simulink model "rate_change_filters_txrx_2ch"  (Simulink 7.7)
settings: Solver=VariableStepDiscrete  SolverMode=SingleTasking  StartTime=0.0  StopTime=1e3  RelTol=1e-3
InitFcn:
  | rate_change_filters_init
StartFcn:
  | rate_change_filters_init
values from neighbouring files (symbols this model uses):
  h32_rs = h32    [rate_change_filters_init.m]
  h64_rs = permute(reshape(h64(1:64),4,4,4),[2 1 3])    [rate_change_filters_init.m]
undefined symbols (not defined in the file or in its folder): gcbh, xlBlockLoadCallback, xlGetNormalizedPeriod
libraries: xbsIndex_r4 x499, simulink x8
(part 3 of 3)

== system rate_change_filters_txrx_2ch/Tx Path/2-Ch Interp A/Adders ==
  In1 : Inport
  In2 : Inport  Port=2
  In3 : Inport  Port=3
  In4 : Inport  Port=4
  In5 : Inport  Port=5
  In6 : Inport  Port=6
  In7 : Inport  Port=7
  In8 : Inport  Port=8
  AddSub{1,3..4,7} (4 alike) : xbsIndex_r4/AddSub  mode=Addition  use_carryin=off  use_carryout=off  en=off  latency=0  precision=Full  arith_type=Unsigned  n_bits=16  bin_pt=14  quantization=Truncate  overflow=Wrap  dbl_ovrd=off  use_behavioral_HDL=off  hw_selection=Fabric  pipelined=off  use_rpm=on  block_type=addsub
      settings: xl_area=[10 0 0 18 0 0 0]  block_version=10.1.3
  AddSub2 : xbsIndex_r4/AddSub  mode=Addition  use_carryin=off  use_carryout=off  en=off  latency=1  precision=Full  arith_type=Unsigned  n_bits=16  bin_pt=14  quantization=Truncate  overflow=Wrap  dbl_ovrd=off  use_behavioral_HDL=off  hw_selection=Fabric  pipelined=off  use_rpm=on  block_type=addsub
      settings: xl_area=[10 20 0 19 0 0 0]  block_version=10.1.3
  AddSub5 : xbsIndex_r4/AddSub  mode=Addition  use_carryin=off  use_carryout=off  en=off  latency=1  precision=Full  arith_type=Unsigned  n_bits=16  bin_pt=14  quantization=Truncate  overflow=Wrap  dbl_ovrd=off  use_behavioral_HDL=off  hw_selection=Fabric  pipelined=off  use_rpm=on  block_type=addsub
      settings: xl_area=[10 20 0 19 0 0 0]  block_version=10.1.3
  AddSub8 : xbsIndex_r4/AddSub  mode=Addition  use_carryin=off  use_carryout=off  en=off  latency=0  precision=User Defined  arith_type="Signed  (2's comp)"  n_bits=16  bin_pt=15  quantization=Truncate  overflow=Flag as error  dbl_ovrd=off  use_behavioral_HDL=off  hw_selection=Fabric  pipelined=off  use_rpm=on  block_type=addsub
      settings: xl_area=[11 0 0 20 0 0 0]  block_version=10.1.3
  Out1 : Outport
  wires:
  AddSub5/1 -> AddSub8/2
  AddSub2/1 -> AddSub8/1
  AddSub4/1 -> AddSub5/2
  AddSub3/1 -> AddSub5/1
  AddSub1/1 -> AddSub2/2
  AddSub7/1 -> AddSub2/1
  In1/1 -> AddSub7/1
  In2/1 -> AddSub7/2
  In3/1 -> AddSub1/1
  In4/1 -> AddSub1/2
  AddSub8/1 -> Out1/1
  In5/1 -> AddSub3/1
  In6/1 -> AddSub3/2
  In7/1 -> AddSub4/1
  In8/1 -> AddSub4/2

== system rate_change_filters_txrx_2ch/Tx Path/2-Ch Interp A/Mults & ROMs ==
  In1 : Inport
  In2 : Inport  Port=2
  In3 : Inport  Port=3
  In4 : Inport  Port=4
  In5 : Inport  Port=5
  In6 : Inport  Port=6
  In7 : Inport  Port=7
  In8 : Inport  Port=8
  Mult{1..8} (8 alike) : xbsIndex_r4/Mult  precision=User Defined  arith_type="Signed  (2's comp)"  n_bits=18  bin_pt=17  quantization=Truncate  overflow=Flag as error  en=off  latency=1  dbl_ovrd=off  use_behavioral_HDL=off  opt=Speed  use_embedded=on  optimum_pipeline=off  pipeline=on  use_rpm=on  placement_style=Triangular  block_type=mult
      settings: infoedit=Hardware notes: To use the internal pipeline stage of the dedicated multiplier you must select 'Pipeline for maximum performance'.  xl_area=[9 -15 0 18 0 1 0]  block_version=10.1.3
  Out1 : Outport
  Out2 : Outport  Port=2
  Out3 : Outport  Port=3
  Out4 : Outport  Port=4
  Out5 : Outport  Port=5
  Out6 : Outport  Port=6
  Out7 : Outport  Port=7
  Out8 : Outport  Port=8
  wires:
  [TX_ROM_7] -> Mult8/2
  [TX_ROM_6] -> Mult7/2
  [TX_ROM_5] -> Mult6/2
  [TX_ROM_4] -> Mult5/2
  [TX_ROM_3] -> Mult4/2
  [TX_ROM_2] -> Mult3/2
  [TX_ROM_1] -> Mult1/2
  [TX_ROM_0] -> Mult2/2
  In1/1 -> Mult2/1
  Mult2/1 -> Out1/1
  In2/1 -> Mult1/1
  Mult1/1 -> Out2/1
  In3/1 -> Mult3/1
  Mult3/1 -> Out3/1
  In4/1 -> Mult4/1
  Mult4/1 -> Out4/1
  In5/1 -> Mult5/1
  Mult5/1 -> Out5/1
  In6/1 -> Mult6/1
  Mult6/1 -> Out6/1
  In7/1 -> Mult7/1
  Mult7/1 -> Out7/1
  In8/1 -> Mult8/1
  Mult8/1 -> Out8/1

== system rate_change_filters_txrx_2ch/Tx Path/2-Ch Interp A/Sample RAMs ==
  A : Inport
  B : Inport  Port=2
  Delays : Subsystem
  Delays1 : Subsystem
  Time Division Multiplexer{1..7,16} (8 alike) : xbsIndex_r4/Time Division Multiplexer  inputs=2  vin=off  dbl_ovrd=off  explicit_period=off  period=1  block_type=tdm
      settings: infoedit="Multiple inputs are sampled and  presented serially at the output."  xl_area=[3 2 0 35 0 0 0]  block_version=10.1.3
  Out1 : Outport
  Out2 : Outport  Port=2
  Out3 : Outport  Port=3
  Out4 : Outport  Port=4
  Out5 : Outport  Port=5
  Out6 : Outport  Port=6
  Out7 : Outport  Port=7
  Out8 : Outport  Port=8
  wires:
  Delays/1(Out1) -> Time Division Multiplexer16/1
  Delays1/1(Out1) -> Time Division Multiplexer16/2
  Delays/2(Out2) -> Time Division Multiplexer1/1
  Delays1/2(Out2) -> Time Division Multiplexer1/2
  Delays/3(Out3) -> Time Division Multiplexer3/1
  Delays/4(Out4) -> Time Division Multiplexer2/1
  Delays/5(Out5) -> Time Division Multiplexer5/1
  Delays/6(Out6) -> Time Division Multiplexer4/1
  Delays/7(Out7) -> Time Division Multiplexer7/1
  Delays/8(Out8) -> Time Division Multiplexer6/1
  Delays1/3(Out3) -> Time Division Multiplexer3/2
  Delays1/4(Out4) -> Time Division Multiplexer2/2
  Delays1/5(Out5) -> Time Division Multiplexer5/2
  Delays1/6(Out6) -> Time Division Multiplexer4/2
  Delays1/7(Out7) -> Time Division Multiplexer7/2
  Delays1/8(Out8) -> Time Division Multiplexer6/2
  Time Division Multiplexer16/1 -> Out1/1
  Time Division Multiplexer1/1 -> Out2/1
  Time Division Multiplexer3/1 -> Out3/1
  Time Division Multiplexer2/1 -> Out4/1
  A/1 -> Delays/1(X)
  Time Division Multiplexer5/1 -> Out5/1
  Time Division Multiplexer4/1 -> Out6/1
  Time Division Multiplexer7/1 -> Out7/1
  Time Division Multiplexer6/1 -> Out8/1
  B/1 -> Delays1/1(X)

== system rate_change_filters_txrx_2ch/Tx Path/2-Ch Interp B/Adders ==
  In1 : Inport
  In2 : Inport  Port=2
  In3 : Inport  Port=3
  In4 : Inport  Port=4
  In5 : Inport  Port=5
  In6 : Inport  Port=6
  In7 : Inport  Port=7
  In8 : Inport  Port=8
  AddSub{1,3..4,7} (4 alike) : xbsIndex_r4/AddSub  mode=Addition  use_carryin=off  use_carryout=off  en=off  latency=0  precision=Full  arith_type=Unsigned  n_bits=16  bin_pt=14  quantization=Truncate  overflow=Wrap  dbl_ovrd=off  use_behavioral_HDL=off  hw_selection=Fabric  pipelined=off  use_rpm=on  block_type=addsub
      settings: xl_area=[10 0 0 18 0 0 0]  block_version=10.1.3
  AddSub2 : xbsIndex_r4/AddSub  mode=Addition  use_carryin=off  use_carryout=off  en=off  latency=1  precision=Full  arith_type=Unsigned  n_bits=16  bin_pt=14  quantization=Truncate  overflow=Wrap  dbl_ovrd=off  use_behavioral_HDL=off  hw_selection=Fabric  pipelined=off  use_rpm=on  block_type=addsub
      settings: xl_area=[10 20 0 19 0 0 0]  block_version=10.1.3
  AddSub5 : xbsIndex_r4/AddSub  mode=Addition  use_carryin=off  use_carryout=off  en=off  latency=1  precision=Full  arith_type=Unsigned  n_bits=16  bin_pt=14  quantization=Truncate  overflow=Wrap  dbl_ovrd=off  use_behavioral_HDL=off  hw_selection=Fabric  pipelined=off  use_rpm=on  block_type=addsub
      settings: xl_area=[10 20 0 19 0 0 0]  block_version=10.1.3
  AddSub8 : xbsIndex_r4/AddSub  mode=Addition  use_carryin=off  use_carryout=off  en=off  latency=0  precision=User Defined  arith_type="Signed  (2's comp)"  n_bits=16  bin_pt=15  quantization=Truncate  overflow=Flag as error  dbl_ovrd=off  use_behavioral_HDL=off  hw_selection=Fabric  pipelined=off  use_rpm=on  block_type=addsub
      settings: xl_area=[11 0 0 20 0 0 0]  block_version=10.1.3
  Out1 : Outport
  wires:
  In8/1 -> AddSub4/2
  In7/1 -> AddSub4/1
  In6/1 -> AddSub3/2
  In5/1 -> AddSub3/1
  AddSub8/1 -> Out1/1
  In4/1 -> AddSub1/2
  In3/1 -> AddSub1/1
  In2/1 -> AddSub7/2
  In1/1 -> AddSub7/1
  AddSub7/1 -> AddSub2/1
  AddSub1/1 -> AddSub2/2
  AddSub3/1 -> AddSub5/1
  AddSub4/1 -> AddSub5/2
  AddSub2/1 -> AddSub8/1
  AddSub5/1 -> AddSub8/2

== system rate_change_filters_txrx_2ch/Tx Path/2-Ch Interp B/Mults & ROMs ==
  In1 : Inport
  In2 : Inport  Port=2
  In3 : Inport  Port=3
  In4 : Inport  Port=4
  In5 : Inport  Port=5
  In6 : Inport  Port=6
  In7 : Inport  Port=7
  In8 : Inport  Port=8
  Mult{1..8} (8 alike) : xbsIndex_r4/Mult  precision=User Defined  arith_type="Signed  (2's comp)"  n_bits=18  bin_pt=17  quantization=Truncate  overflow=Flag as error  en=off  latency=1  dbl_ovrd=off  use_behavioral_HDL=off  opt=Speed  use_embedded=on  optimum_pipeline=off  pipeline=on  use_rpm=on  placement_style=Triangular  block_type=mult
      settings: infoedit=Hardware notes: To use the internal pipeline stage of the dedicated multiplier you must select 'Pipeline for maximum performance'.  xl_area=[9 -15 0 18 0 1 0]  block_version=10.1.3
  Out1 : Outport
  Out2 : Outport  Port=2
  Out3 : Outport  Port=3
  Out4 : Outport  Port=4
  Out5 : Outport  Port=5
  Out6 : Outport  Port=6
  Out7 : Outport  Port=7
  Out8 : Outport  Port=8
  wires:
  Mult8/1 -> Out8/1
  In8/1 -> Mult8/1
  Mult7/1 -> Out7/1
  In7/1 -> Mult7/1
  Mult6/1 -> Out6/1
  In6/1 -> Mult6/1
  Mult5/1 -> Out5/1
  In5/1 -> Mult5/1
  Mult4/1 -> Out4/1
  In4/1 -> Mult4/1
  Mult3/1 -> Out3/1
  In3/1 -> Mult3/1
  Mult1/1 -> Out2/1
  In2/1 -> Mult1/1
  Mult2/1 -> Out1/1
  In1/1 -> Mult2/1
  [TX_ROM_0] -> Mult2/2
  [TX_ROM_1] -> Mult1/2
  [TX_ROM_2] -> Mult3/2
  [TX_ROM_3] -> Mult4/2
  [TX_ROM_4] -> Mult5/2
  [TX_ROM_5] -> Mult6/2
  [TX_ROM_6] -> Mult7/2
  [TX_ROM_7] -> Mult8/2

== system rate_change_filters_txrx_2ch/Tx Path/2-Ch Interp B/Sample RAMs ==
  A : Inport
  B : Inport  Port=2
  Delays : Subsystem
  Delays1 : Subsystem
  Time Division Multiplexer{1..7,16} (8 alike) : xbsIndex_r4/Time Division Multiplexer  inputs=2  vin=off  dbl_ovrd=off  explicit_period=off  period=1  block_type=tdm
      settings: infoedit="Multiple inputs are sampled and  presented serially at the output."  xl_area=[3 2 0 35 0 0 0]  block_version=10.1.3
  Out1 : Outport
  Out2 : Outport  Port=2
  Out3 : Outport  Port=3
  Out4 : Outport  Port=4
  Out5 : Outport  Port=5
  Out6 : Outport  Port=6
  Out7 : Outport  Port=7
  Out8 : Outport  Port=8
  wires:
  B/1 -> Delays1/1(X)
  Time Division Multiplexer6/1 -> Out8/1
  Time Division Multiplexer7/1 -> Out7/1
  Time Division Multiplexer4/1 -> Out6/1
  Time Division Multiplexer5/1 -> Out5/1
  A/1 -> Delays/1(X)
  Time Division Multiplexer2/1 -> Out4/1
  Time Division Multiplexer3/1 -> Out3/1
  Time Division Multiplexer1/1 -> Out2/1
  Time Division Multiplexer16/1 -> Out1/1
  Delays1/8(Out8) -> Time Division Multiplexer6/2
  Delays1/7(Out7) -> Time Division Multiplexer7/2
  Delays1/6(Out6) -> Time Division Multiplexer4/2
  Delays1/5(Out5) -> Time Division Multiplexer5/2
  Delays1/4(Out4) -> Time Division Multiplexer2/2
  Delays1/3(Out3) -> Time Division Multiplexer3/2
  Delays/8(Out8) -> Time Division Multiplexer6/1
  Delays/7(Out7) -> Time Division Multiplexer7/1
  Delays/6(Out6) -> Time Division Multiplexer4/1
  Delays/5(Out5) -> Time Division Multiplexer5/1
  Delays/4(Out4) -> Time Division Multiplexer2/1
  Delays/3(Out3) -> Time Division Multiplexer3/1
  Delays1/2(Out2) -> Time Division Multiplexer1/2
  Delays/2(Out2) -> Time Division Multiplexer1/1
  Delays1/1(Out1) -> Time Division Multiplexer16/2
  Delays/1(Out1) -> Time Division Multiplexer16/1

== system rate_change_filters_txrx_2ch/Rx Path/2-Ch Decimation A/Adders/Adder Tree ==
  In1 : Inport
  In2 : Inport  Port=2
  In3 : Inport  Port=3
  In4 : Inport  Port=4
  In5 : Inport  Port=5
  In6 : Inport  Port=6
  In7 : Inport  Port=7
  In8 : Inport  Port=8
  AddSub{,1,3..4} (4 alike) : xbsIndex_r4/AddSub  mode=Addition  use_carryin=off  use_carryout=off  en=off  latency=0  precision=Full  arith_type=Unsigned  n_bits=8  bin_pt=2  quantization=Truncate  overflow=Wrap  dbl_ovrd=off  use_behavioral_HDL=on  hw_selection=Fabric  pipelined=off  use_rpm=on  block_type=addsub
      settings: xl_area=[13 0 0 25 0 0 0]  block_version=9.1.01
  AddSub2 : xbsIndex_r4/AddSub  mode=Addition  use_carryin=off  use_carryout=off  en=off  latency=1  precision=Full  arith_type=Unsigned  n_bits=8  bin_pt=2  quantization=Truncate  overflow=Wrap  dbl_ovrd=off  use_behavioral_HDL=on  hw_selection=Fabric  pipelined=off  use_rpm=on  block_type=addsub
      settings: xl_area=[14 0 0 26 0 0 0]  block_version=9.1.01
  AddSub5 : xbsIndex_r4/AddSub  mode=Addition  use_carryin=off  use_carryout=off  en=off  latency=1  precision=Full  arith_type=Unsigned  n_bits=8  bin_pt=2  quantization=Truncate  overflow=Wrap  dbl_ovrd=off  use_behavioral_HDL=on  hw_selection=Fabric  pipelined=off  use_rpm=on  block_type=addsub
      settings: xl_area=[14 0 0 26 0 0 0]  block_version=9.1.01
  AddSub6 : xbsIndex_r4/AddSub  mode=Addition  use_carryin=off  use_carryout=off  en=off  latency=0  precision=Full  arith_type="Signed  (2's comp)"  n_bits=1  bin_pt=0  quantization=Truncate  overflow=Flag as error  dbl_ovrd=off  use_behavioral_HDL=on  hw_selection=Fabric  pipelined=off  use_rpm=on  block_type=addsub
      settings: xl_area=[14 0 0 27 0 0 0]  block_version=9.1.01
  Out1 : Outport
  wires:
  In8/1 -> AddSub4/2
  In7/1 -> AddSub4/1
  In6/1 -> AddSub3/2
  In5/1 -> AddSub3/1
  AddSub6/1 -> Out1/1
  In4/1 -> AddSub1/2
  In3/1 -> AddSub1/1
  In2/1 -> AddSub/2
  In1/1 -> AddSub/1
  AddSub/1 -> AddSub2/1
  AddSub1/1 -> AddSub2/2
  AddSub3/1 -> AddSub5/1
  AddSub4/1 -> AddSub5/2
  AddSub2/1 -> AddSub6/1
  AddSub5/1 -> AddSub6/2

== system rate_change_filters_txrx_2ch/Rx Path/2-Ch Decimation A/Adders/Adder Tree1 ==
  In1 : Inport
  In2 : Inport  Port=2
  In3 : Inport  Port=3
  In4 : Inport  Port=4
  In5 : Inport  Port=5
  In6 : Inport  Port=6
  In7 : Inport  Port=7
  In8 : Inport  Port=8
  AddSub{,1,3..4} (4 alike) : xbsIndex_r4/AddSub  mode=Addition  use_carryin=off  use_carryout=off  en=off  latency=0  precision=Full  arith_type=Unsigned  n_bits=8  bin_pt=2  quantization=Truncate  overflow=Wrap  dbl_ovrd=off  use_behavioral_HDL=on  hw_selection=Fabric  pipelined=off  use_rpm=on  block_type=addsub
      settings: xl_area=[13 0 0 25 0 0 0]  block_version=9.1.01
  AddSub2 : xbsIndex_r4/AddSub  mode=Addition  use_carryin=off  use_carryout=off  en=off  latency=1  precision=Full  arith_type=Unsigned  n_bits=8  bin_pt=2  quantization=Truncate  overflow=Wrap  dbl_ovrd=off  use_behavioral_HDL=on  hw_selection=Fabric  pipelined=off  use_rpm=on  block_type=addsub
      settings: xl_area=[14 0 0 26 0 0 0]  block_version=9.1.01
  AddSub5 : xbsIndex_r4/AddSub  mode=Addition  use_carryin=off  use_carryout=off  en=off  latency=1  precision=Full  arith_type=Unsigned  n_bits=8  bin_pt=2  quantization=Truncate  overflow=Wrap  dbl_ovrd=off  use_behavioral_HDL=on  hw_selection=Fabric  pipelined=off  use_rpm=on  block_type=addsub
      settings: xl_area=[14 0 0 26 0 0 0]  block_version=9.1.01
  AddSub6 : xbsIndex_r4/AddSub  mode=Addition  use_carryin=off  use_carryout=off  en=off  latency=0  precision=Full  arith_type="Signed  (2's comp)"  n_bits=1  bin_pt=0  quantization=Truncate  overflow=Flag as error  dbl_ovrd=off  use_behavioral_HDL=on  hw_selection=Fabric  pipelined=off  use_rpm=on  block_type=addsub
      settings: xl_area=[14 0 0 27 0 0 0]  block_version=9.1.01
  Out1 : Outport
  wires:
  AddSub5/1 -> AddSub6/2
  AddSub2/1 -> AddSub6/1
  AddSub4/1 -> AddSub5/2
  AddSub3/1 -> AddSub5/1
  AddSub1/1 -> AddSub2/2
  AddSub/1 -> AddSub2/1
  In1/1 -> AddSub/1
  In2/1 -> AddSub/2
  In3/1 -> AddSub1/1
  In4/1 -> AddSub1/2
  AddSub6/1 -> Out1/1
  In5/1 -> AddSub3/1
  In6/1 -> AddSub3/2
  In7/1 -> AddSub4/1
  In8/1 -> AddSub4/2

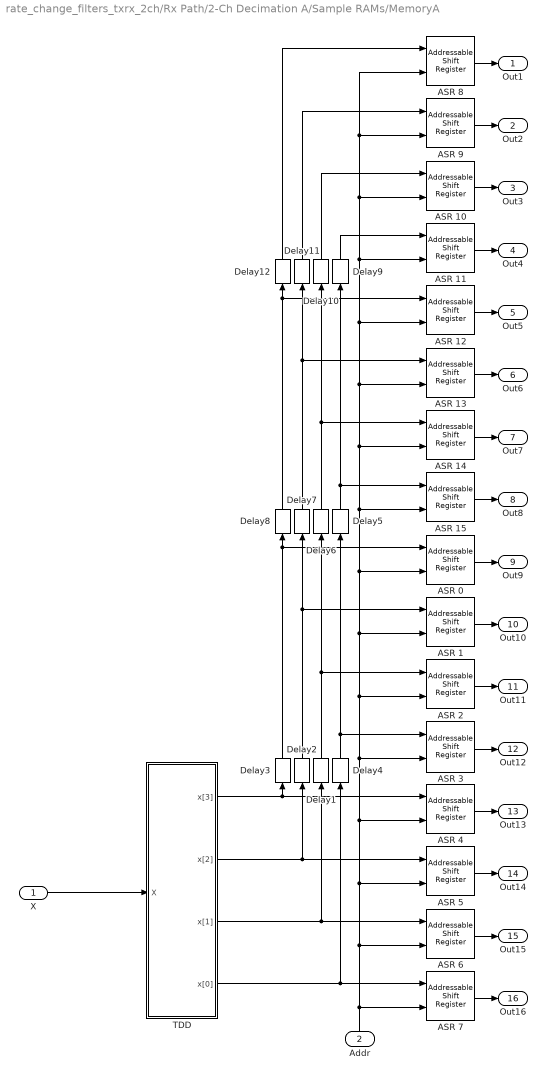
== system rate_change_filters_txrx_2ch/Rx Path/2-Ch Decimation A/Sample RAMs/MemoryA ==
  X : Inport
  Addr : Inport  Port=2
  ASR {0..15} (16 alike) : xbsIndex_r4/Addressable Shift Register  infer_latency=on  depth=2  initVector=[0]  en=off  dbl_ovrd=off  use_behavioral_HDL=off  Optimization=Resource  use_rpm=on  block_type=addrsr
      settings: xl_area=[7 0 0 14 0 0 0]  block_version=9.1.01
      settings: infoedit=|
      | Delay of  configurable length.  Any element  in the delay
      |     line   can    be   addressed   and   driven    onto   the   output
      |     port.<P><P>Hardware  notes: Implemented  using SRL16s.
      |     If Virtex-4, Virtex-II or Spartan-3 devices are used, multiple SRLC16s are cascaded together.
  Delay{1..12} (12 alike) : xbsIndex_r4/Delay  rst=off  infoeditControl=Selection of Reset will increase slice count due to use of real FFs and instead of SRLs  en=off  latency=4  dbl_ovrd=off  reg_retiming=off  block_type=delay
      settings: xl_area=[7 14 0 14 0 0 0]  block_version=9.1.01
  TDD : Subsystem
  Out1 : Outport
  Out2 : Outport  Port=2
  Out3 : Outport  Port=3
  Out4 : Outport  Port=4
  Out5 : Outport  Port=5
  Out6 : Outport  Port=6
  Out7 : Outport  Port=7
  Out8 : Outport  Port=8
  Out9 : Outport  Port=9
  Out10 : Outport  Port=10
  Out11 : Outport  Port=11
  Out12 : Outport  Port=12
  Out13 : Outport  Port=13
  Out14 : Outport  Port=14
  Out15 : Outport  Port=15
  Out16 : Outport  Port=16
  wires:
  X/1 -> TDD/1(X)
  TDD/2(x[2]) -> ASR 5/1, Delay2/1
  TDD/1(x[3]) -> ASR 4/1, Delay3/1
  TDD/4(x[0]) -> ASR 7/1, Delay4/1
  Delay12/1 -> ASR 8/1
  Delay11/1 -> ASR 9/1
  Delay10/1 -> ASR 10/1
  Delay9/1 -> ASR 11/1
  Delay8/1 -> Delay12/1, ASR 12/1
  Delay7/1 -> Delay11/1, ASR 13/1
  Delay6/1 -> Delay10/1, ASR 14/1
  Delay5/1 -> Delay9/1, ASR 15/1
  TDD/3(x[1]) -> ASR 6/1, Delay1/1
  Addr/1 -> ASR 7/2, ASR 6/2, ASR 5/2, ASR 4/2, ASR 3/2, ASR 2/2, ASR 1/2, ASR 0/2, ASR 15/2, ASR 14/2, ASR 13/2, ASR 12/2, ASR 11/2, ASR 10/2, ASR 8/2, ASR 9/2
  Delay3/1 -> ASR 0/1, Delay8/1
  Delay2/1 -> ASR 1/1, Delay7/1
  Delay1/1 -> ASR 2/1, Delay6/1
  Delay4/1 -> ASR 3/1, Delay5/1
  ASR 8/1 -> Out1/1
  ASR 9/1 -> Out2/1
  ASR 10/1 -> Out3/1
  ASR 11/1 -> Out4/1
  ASR 12/1 -> Out5/1
  ASR 13/1 -> Out6/1
  ASR 14/1 -> Out7/1
  ASR 15/1 -> Out8/1
  ASR 0/1 -> Out9/1
  ASR 1/1 -> Out10/1
  ASR 2/1 -> Out11/1
  ASR 3/1 -> Out12/1
  ASR 4/1 -> Out13/1
  ASR 5/1 -> Out14/1
  ASR 6/1 -> Out15/1
  ASR 7/1 -> Out16/1

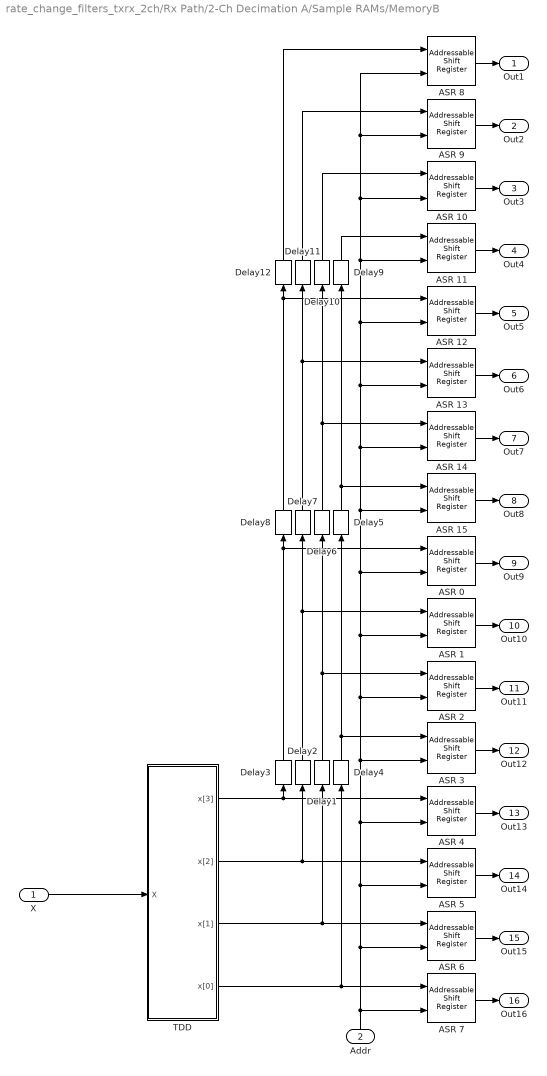
== system rate_change_filters_txrx_2ch/Rx Path/2-Ch Decimation A/Sample RAMs/MemoryB ==
  X : Inport
  Addr : Inport  Port=2
  ASR {0..15} (16 alike) : xbsIndex_r4/Addressable Shift Register  infer_latency=on  depth=2  initVector=[0]  en=off  dbl_ovrd=off  use_behavioral_HDL=off  Optimization=Resource  use_rpm=on  block_type=addrsr
      settings: xl_area=[7 0 0 14 0 0 0]  block_version=9.1.01
      settings: infoedit=|
      | Delay of  configurable length.  Any element  in the delay
      |     line   can    be   addressed   and   driven    onto   the   output
      |     port.<P><P>Hardware  notes: Implemented  using SRL16s.
      |     If Virtex-4, Virtex-II or Spartan-3 devices are used, multiple SRLC16s are cascaded together.
  Delay{1..12} (12 alike) : xbsIndex_r4/Delay  rst=off  infoeditControl=Selection of Reset will increase slice count due to use of real FFs and instead of SRLs  en=off  latency=4  dbl_ovrd=off  reg_retiming=off  block_type=delay
      settings: xl_area=[7 14 0 14 0 0 0]  block_version=9.1.01
  TDD : Subsystem
  Out1 : Outport
  Out2 : Outport  Port=2
  Out3 : Outport  Port=3
  Out4 : Outport  Port=4
  Out5 : Outport  Port=5
  Out6 : Outport  Port=6
  Out7 : Outport  Port=7
  Out8 : Outport  Port=8
  Out9 : Outport  Port=9
  Out10 : Outport  Port=10
  Out11 : Outport  Port=11
  Out12 : Outport  Port=12
  Out13 : Outport  Port=13
  Out14 : Outport  Port=14
  Out15 : Outport  Port=15
  Out16 : Outport  Port=16
  wires:
  ASR 7/1 -> Out16/1
  ASR 6/1 -> Out15/1
  ASR 5/1 -> Out14/1
  ASR 4/1 -> Out13/1
  ASR 3/1 -> Out12/1
  ASR 2/1 -> Out11/1
  ASR 1/1 -> Out10/1
  ASR 0/1 -> Out9/1
  ASR 15/1 -> Out8/1
  ASR 14/1 -> Out7/1
  ASR 13/1 -> Out6/1
  ASR 12/1 -> Out5/1
  ASR 11/1 -> Out4/1
  ASR 10/1 -> Out3/1
  ASR 9/1 -> Out2/1
  ASR 8/1 -> Out1/1
  Delay4/1 -> Delay5/1, ASR 3/1
  Delay1/1 -> Delay6/1, ASR 2/1
  Delay2/1 -> Delay7/1, ASR 1/1
  Delay3/1 -> Delay8/1, ASR 0/1
  Addr/1 -> ASR 9/2, ASR 8/2, ASR 10/2, ASR 11/2, ASR 12/2, ASR 13/2, ASR 14/2, ASR 15/2, ASR 0/2, ASR 1/2, ASR 2/2, ASR 3/2, ASR 4/2, ASR 5/2, ASR 6/2, ASR 7/2
  TDD/3(x[1]) -> Delay1/1, ASR 6/1
  Delay5/1 -> ASR 15/1, Delay9/1
  Delay6/1 -> ASR 14/1, Delay10/1
  Delay7/1 -> ASR 13/1, Delay11/1
  Delay8/1 -> ASR 12/1, Delay12/1
  Delay9/1 -> ASR 11/1
  Delay10/1 -> ASR 10/1
  Delay11/1 -> ASR 9/1
  Delay12/1 -> ASR 8/1
  TDD/4(x[0]) -> Delay4/1, ASR 7/1
  TDD/1(x[3]) -> Delay3/1, ASR 4/1
  TDD/2(x[2]) -> Delay2/1, ASR 5/1
  X/1 -> TDD/1(X)

== system rate_change_filters_txrx_2ch/Rx Path/2-Ch Decimation B/Adders/Adder Tree ==
  In1 : Inport
  In2 : Inport  Port=2
  In3 : Inport  Port=3
  In4 : Inport  Port=4
  In5 : Inport  Port=5
  In6 : Inport  Port=6
  In7 : Inport  Port=7
  In8 : Inport  Port=8
  AddSub{,1,3..4} (4 alike) : xbsIndex_r4/AddSub  mode=Addition  use_carryin=off  use_carryout=off  en=off  latency=0  precision=Full  arith_type=Unsigned  n_bits=8  bin_pt=2  quantization=Truncate  overflow=Wrap  dbl_ovrd=off  use_behavioral_HDL=on  hw_selection=Fabric  pipelined=off  use_rpm=on  block_type=addsub
      settings: xl_area=[13 0 0 25 0 0 0]  block_version=9.1.01
  AddSub2 : xbsIndex_r4/AddSub  mode=Addition  use_carryin=off  use_carryout=off  en=off  latency=1  precision=Full  arith_type=Unsigned  n_bits=8  bin_pt=2  quantization=Truncate  overflow=Wrap  dbl_ovrd=off  use_behavioral_HDL=on  hw_selection=Fabric  pipelined=off  use_rpm=on  block_type=addsub
      settings: xl_area=[14 0 0 26 0 0 0]  block_version=9.1.01
  AddSub5 : xbsIndex_r4/AddSub  mode=Addition  use_carryin=off  use_carryout=off  en=off  latency=1  precision=Full  arith_type=Unsigned  n_bits=8  bin_pt=2  quantization=Truncate  overflow=Wrap  dbl_ovrd=off  use_behavioral_HDL=on  hw_selection=Fabric  pipelined=off  use_rpm=on  block_type=addsub
      settings: xl_area=[14 0 0 26 0 0 0]  block_version=9.1.01
  AddSub6 : xbsIndex_r4/AddSub  mode=Addition  use_carryin=off  use_carryout=off  en=off  latency=0  precision=Full  arith_type="Signed  (2's comp)"  n_bits=1  bin_pt=0  quantization=Truncate  overflow=Flag as error  dbl_ovrd=off  use_behavioral_HDL=on  hw_selection=Fabric  pipelined=off  use_rpm=on  block_type=addsub
      settings: xl_area=[14 0 0 27 0 0 0]  block_version=9.1.01
  Out1 : Outport
  wires:
  AddSub5/1 -> AddSub6/2
  AddSub2/1 -> AddSub6/1
  AddSub4/1 -> AddSub5/2
  AddSub3/1 -> AddSub5/1
  AddSub1/1 -> AddSub2/2
  AddSub/1 -> AddSub2/1
  In1/1 -> AddSub/1
  In2/1 -> AddSub/2
  In3/1 -> AddSub1/1
  In4/1 -> AddSub1/2
  AddSub6/1 -> Out1/1
  In5/1 -> AddSub3/1
  In6/1 -> AddSub3/2
  In7/1 -> AddSub4/1
  In8/1 -> AddSub4/2

== system rate_change_filters_txrx_2ch/Rx Path/2-Ch Decimation B/Adders/Adder Tree1 ==
  In1 : Inport
  In2 : Inport  Port=2
  In3 : Inport  Port=3
  In4 : Inport  Port=4
  In5 : Inport  Port=5
  In6 : Inport  Port=6
  In7 : Inport  Port=7
  In8 : Inport  Port=8
  AddSub{,1,3..4} (4 alike) : xbsIndex_r4/AddSub  mode=Addition  use_carryin=off  use_carryout=off  en=off  latency=0  precision=Full  arith_type=Unsigned  n_bits=8  bin_pt=2  quantization=Truncate  overflow=Wrap  dbl_ovrd=off  use_behavioral_HDL=on  hw_selection=Fabric  pipelined=off  use_rpm=on  block_type=addsub
      settings: xl_area=[13 0 0 25 0 0 0]  block_version=9.1.01
  AddSub2 : xbsIndex_r4/AddSub  mode=Addition  use_carryin=off  use_carryout=off  en=off  latency=1  precision=Full  arith_type=Unsigned  n_bits=8  bin_pt=2  quantization=Truncate  overflow=Wrap  dbl_ovrd=off  use_behavioral_HDL=on  hw_selection=Fabric  pipelined=off  use_rpm=on  block_type=addsub
      settings: xl_area=[14 0 0 26 0 0 0]  block_version=9.1.01
  AddSub5 : xbsIndex_r4/AddSub  mode=Addition  use_carryin=off  use_carryout=off  en=off  latency=1  precision=Full  arith_type=Unsigned  n_bits=8  bin_pt=2  quantization=Truncate  overflow=Wrap  dbl_ovrd=off  use_behavioral_HDL=on  hw_selection=Fabric  pipelined=off  use_rpm=on  block_type=addsub
      settings: xl_area=[14 0 0 26 0 0 0]  block_version=9.1.01
  AddSub6 : xbsIndex_r4/AddSub  mode=Addition  use_carryin=off  use_carryout=off  en=off  latency=0  precision=Full  arith_type="Signed  (2's comp)"  n_bits=1  bin_pt=0  quantization=Truncate  overflow=Flag as error  dbl_ovrd=off  use_behavioral_HDL=on  hw_selection=Fabric  pipelined=off  use_rpm=on  block_type=addsub
      settings: xl_area=[14 0 0 27 0 0 0]  block_version=9.1.01
  Out1 : Outport
  wires:
  In8/1 -> AddSub4/2
  In7/1 -> AddSub4/1
  In6/1 -> AddSub3/2
  In5/1 -> AddSub3/1
  AddSub6/1 -> Out1/1
  In4/1 -> AddSub1/2
  In3/1 -> AddSub1/1
  In2/1 -> AddSub/2
  In1/1 -> AddSub/1
  AddSub/1 -> AddSub2/1
  AddSub1/1 -> AddSub2/2
  AddSub3/1 -> AddSub5/1
  AddSub4/1 -> AddSub5/2
  AddSub2/1 -> AddSub6/1
  AddSub5/1 -> AddSub6/2

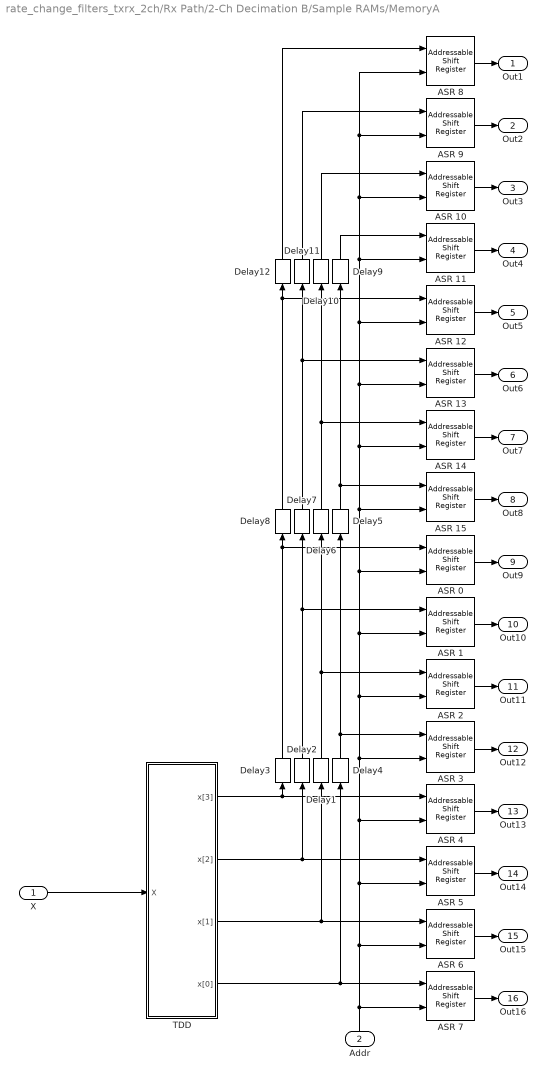
== system rate_change_filters_txrx_2ch/Rx Path/2-Ch Decimation B/Sample RAMs/MemoryA ==
  X : Inport
  Addr : Inport  Port=2
  ASR {0..15} (16 alike) : xbsIndex_r4/Addressable Shift Register  infer_latency=on  depth=2  initVector=[0]  en=off  dbl_ovrd=off  use_behavioral_HDL=off  Optimization=Resource  use_rpm=on  block_type=addrsr
      settings: xl_area=[7 0 0 14 0 0 0]  block_version=9.1.01
      settings: infoedit=|
      | Delay of  configurable length.  Any element  in the delay
      |     line   can    be   addressed   and   driven    onto   the   output
      |     port.<P><P>Hardware  notes: Implemented  using SRL16s.
      |     If Virtex-4, Virtex-II or Spartan-3 devices are used, multiple SRLC16s are cascaded together.
  Delay{1..12} (12 alike) : xbsIndex_r4/Delay  rst=off  infoeditControl=Selection of Reset will increase slice count due to use of real FFs and instead of SRLs  en=off  latency=4  dbl_ovrd=off  reg_retiming=off  block_type=delay
      settings: xl_area=[7 14 0 14 0 0 0]  block_version=9.1.01
  TDD : Subsystem
  Out1 : Outport
  Out2 : Outport  Port=2
  Out3 : Outport  Port=3
  Out4 : Outport  Port=4
  Out5 : Outport  Port=5
  Out6 : Outport  Port=6
  Out7 : Outport  Port=7
  Out8 : Outport  Port=8
  Out9 : Outport  Port=9
  Out10 : Outport  Port=10
  Out11 : Outport  Port=11
  Out12 : Outport  Port=12
  Out13 : Outport  Port=13
  Out14 : Outport  Port=14
  Out15 : Outport  Port=15
  Out16 : Outport  Port=16
  wires:
  ASR 7/1 -> Out16/1
  ASR 6/1 -> Out15/1
  ASR 5/1 -> Out14/1
  ASR 4/1 -> Out13/1
  ASR 3/1 -> Out12/1
  ASR 2/1 -> Out11/1
  ASR 1/1 -> Out10/1
  ASR 0/1 -> Out9/1
  ASR 15/1 -> Out8/1
  ASR 14/1 -> Out7/1
  ASR 13/1 -> Out6/1
  ASR 12/1 -> Out5/1
  ASR 11/1 -> Out4/1
  ASR 10/1 -> Out3/1
  ASR 9/1 -> Out2/1
  ASR 8/1 -> Out1/1
  Delay4/1 -> Delay5/1, ASR 3/1
  Delay1/1 -> Delay6/1, ASR 2/1
  Delay2/1 -> Delay7/1, ASR 1/1
  Delay3/1 -> Delay8/1, ASR 0/1
  Addr/1 -> ASR 9/2, ASR 8/2, ASR 10/2, ASR 11/2, ASR 12/2, ASR 13/2, ASR 14/2, ASR 15/2, ASR 0/2, ASR 1/2, ASR 2/2, ASR 3/2, ASR 4/2, ASR 5/2, ASR 6/2, ASR 7/2
  TDD/3(x[1]) -> Delay1/1, ASR 6/1
  Delay5/1 -> ASR 15/1, Delay9/1
  Delay6/1 -> ASR 14/1, Delay10/1
  Delay7/1 -> ASR 13/1, Delay11/1
  Delay8/1 -> ASR 12/1, Delay12/1
  Delay9/1 -> ASR 11/1
  Delay10/1 -> ASR 10/1
  Delay11/1 -> ASR 9/1
  Delay12/1 -> ASR 8/1
  TDD/4(x[0]) -> Delay4/1, ASR 7/1
  TDD/1(x[3]) -> Delay3/1, ASR 4/1
  TDD/2(x[2]) -> Delay2/1, ASR 5/1
  X/1 -> TDD/1(X)

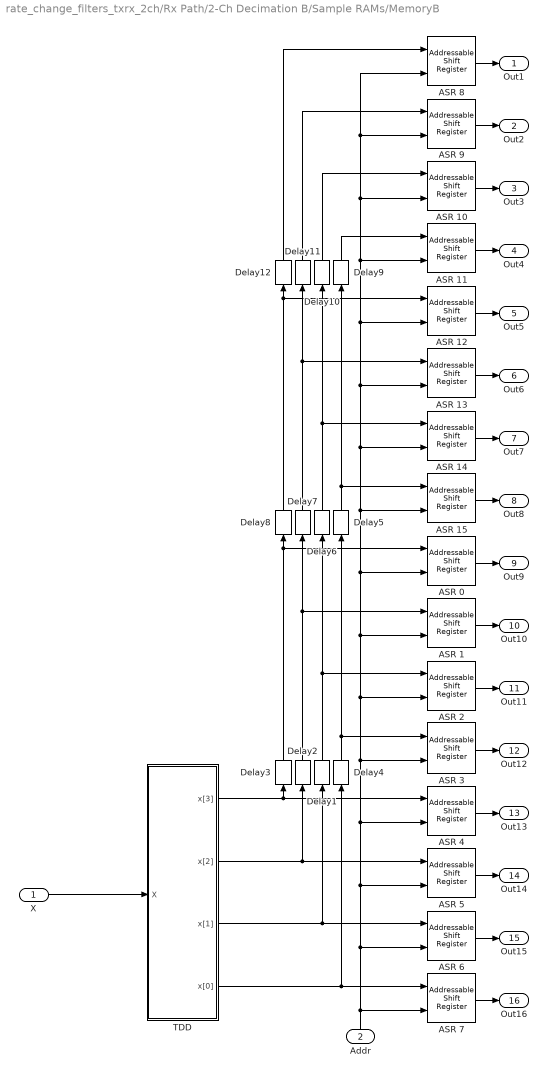
== system rate_change_filters_txrx_2ch/Rx Path/2-Ch Decimation B/Sample RAMs/MemoryB ==
  X : Inport
  Addr : Inport  Port=2
  ASR {0..15} (16 alike) : xbsIndex_r4/Addressable Shift Register  infer_latency=on  depth=2  initVector=[0]  en=off  dbl_ovrd=off  use_behavioral_HDL=off  Optimization=Resource  use_rpm=on  block_type=addrsr
      settings: xl_area=[7 0 0 14 0 0 0]  block_version=9.1.01
      settings: infoedit=|
      | Delay of  configurable length.  Any element  in the delay
      |     line   can    be   addressed   and   driven    onto   the   output
      |     port.<P><P>Hardware  notes: Implemented  using SRL16s.
      |     If Virtex-4, Virtex-II or Spartan-3 devices are used, multiple SRLC16s are cascaded together.
  Delay{1..12} (12 alike) : xbsIndex_r4/Delay  rst=off  infoeditControl=Selection of Reset will increase slice count due to use of real FFs and instead of SRLs  en=off  latency=4  dbl_ovrd=off  reg_retiming=off  block_type=delay
      settings: xl_area=[7 14 0 14 0 0 0]  block_version=9.1.01
  TDD : Subsystem
  Out1 : Outport
  Out2 : Outport  Port=2
  Out3 : Outport  Port=3
  Out4 : Outport  Port=4
  Out5 : Outport  Port=5
  Out6 : Outport  Port=6
  Out7 : Outport  Port=7
  Out8 : Outport  Port=8
  Out9 : Outport  Port=9
  Out10 : Outport  Port=10
  Out11 : Outport  Port=11
  Out12 : Outport  Port=12
  Out13 : Outport  Port=13
  Out14 : Outport  Port=14
  Out15 : Outport  Port=15
  Out16 : Outport  Port=16
  wires:
  X/1 -> TDD/1(X)
  TDD/2(x[2]) -> ASR 5/1, Delay2/1
  TDD/1(x[3]) -> ASR 4/1, Delay3/1
  TDD/4(x[0]) -> ASR 7/1, Delay4/1
  Delay12/1 -> ASR 8/1
  Delay11/1 -> ASR 9/1
  Delay10/1 -> ASR 10/1
  Delay9/1 -> ASR 11/1
  Delay8/1 -> Delay12/1, ASR 12/1
  Delay7/1 -> Delay11/1, ASR 13/1
  Delay6/1 -> Delay10/1, ASR 14/1
  Delay5/1 -> Delay9/1, ASR 15/1
  TDD/3(x[1]) -> ASR 6/1, Delay1/1
  Addr/1 -> ASR 7/2, ASR 6/2, ASR 5/2, ASR 4/2, ASR 3/2, ASR 2/2, ASR 1/2, ASR 0/2, ASR 15/2, ASR 14/2, ASR 13/2, ASR 12/2, ASR 11/2, ASR 10/2, ASR 8/2, ASR 9/2
  Delay3/1 -> ASR 0/1, Delay8/1
  Delay2/1 -> ASR 1/1, Delay7/1
  Delay1/1 -> ASR 2/1, Delay6/1
  Delay4/1 -> ASR 3/1, Delay5/1
  ASR 8/1 -> Out1/1
  ASR 9/1 -> Out2/1
  ASR 10/1 -> Out3/1
  ASR 11/1 -> Out4/1
  ASR 12/1 -> Out5/1
  ASR 13/1 -> Out6/1
  ASR 14/1 -> Out7/1
  ASR 15/1 -> Out8/1
  ASR 0/1 -> Out9/1
  ASR 1/1 -> Out10/1
  ASR 2/1 -> Out11/1
  ASR 3/1 -> Out12/1
  ASR 4/1 -> Out13/1
  ASR 5/1 -> Out14/1
  ASR 6/1 -> Out15/1
  ASR 7/1 -> Out16/1

== system rate_change_filters_txrx_2ch/Tx Path/2-Ch Interp A/Sample RAMs/Delays ==
  X : Inport
  Delay{,1..6} (7 alike) : xbsIndex_r4/Delay  rst=off  infoeditControl=Selection of Reset will increase slice count due to use of real FFs and instead of SRLs  en=off  latency=1  dbl_ovrd=off  reg_retiming=off  block_type=delay
      settings: xl_area=[8 16 0 0 0 0 0]
  Up Sample{1..6,10,15} (8 alike) : xbsIndex_r4/Up Sample  sample_ratio=4  copy_samples=on  en=off  latency=0  dbl_ovrd=off  block_type=usamp
      settings: infoedit="Up samples input data.  Inserted values  can be zeros or copies of the most recent input sample.<P><P>Hardware notes: No hardware is needed if inserted values are copies of the input sample; otherwise, a mux and single bit flip-flop are used."  xl_area=[0 0 0 0 0 0 0]  block_version=10.1.3
  Out1 : Outport
  Out2 : Outport  Port=2
  Out3 : Outport  Port=3
  Out4 : Outport  Port=4
  Out5 : Outport  Port=5
  Out6 : Outport  Port=6
  Out7 : Outport  Port=7
  Out8 : Outport  Port=8
  wires:
  X/1 -> Delay/1, Up Sample2/1
  Delay6/1 -> Up Sample15/1
  Delay5/1 -> Delay6/1, Up Sample6/1
  Delay4/1 -> Delay5/1, Up Sample5/1
  Delay3/1 -> Delay4/1, Up Sample4/1
  Delay2/1 -> Delay3/1, Up Sample3/1
  Delay1/1 -> Delay2/1, Up Sample10/1
  Delay/1 -> Delay1/1, Up Sample1/1
  Up Sample2/1 -> Out1/1
  Up Sample1/1 -> Out2/1
  Up Sample10/1 -> Out3/1
  Up Sample3/1 -> Out4/1
  Up Sample4/1 -> Out5/1
  Up Sample5/1 -> Out6/1
  Up Sample6/1 -> Out7/1
  Up Sample15/1 -> Out8/1

== system rate_change_filters_txrx_2ch/Tx Path/2-Ch Interp A/Sample RAMs/Delays1 ==
  X : Inport
  Delay{,1..6} (7 alike) : xbsIndex_r4/Delay  rst=off  infoeditControl=Selection of Reset will increase slice count due to use of real FFs and instead of SRLs  en=off  latency=1  dbl_ovrd=off  reg_retiming=off  block_type=delay
      settings: xl_area=[8 16 0 0 0 0 0]
  Up Sample{1..6,10,15} (8 alike) : xbsIndex_r4/Up Sample  sample_ratio=4  copy_samples=on  en=off  latency=0  dbl_ovrd=off  block_type=usamp
      settings: infoedit="Up samples input data.  Inserted values  can be zeros or copies of the most recent input sample.<P><P>Hardware notes: No hardware is needed if inserted values are copies of the input sample; otherwise, a mux and single bit flip-flop are used."  xl_area=[0 0 0 0 0 0 0]  block_version=10.1.3
  Out1 : Outport
  Out2 : Outport  Port=2
  Out3 : Outport  Port=3
  Out4 : Outport  Port=4
  Out5 : Outport  Port=5
  Out6 : Outport  Port=6
  Out7 : Outport  Port=7
  Out8 : Outport  Port=8
  wires:
  Up Sample15/1 -> Out8/1
  Up Sample6/1 -> Out7/1
  Up Sample5/1 -> Out6/1
  Up Sample4/1 -> Out5/1
  Up Sample3/1 -> Out4/1
  Up Sample10/1 -> Out3/1
  Up Sample1/1 -> Out2/1
  Up Sample2/1 -> Out1/1
  Delay/1 -> Up Sample1/1, Delay1/1
  Delay1/1 -> Up Sample10/1, Delay2/1
  Delay2/1 -> Up Sample3/1, Delay3/1
  Delay3/1 -> Up Sample4/1, Delay4/1
  Delay4/1 -> Up Sample5/1, Delay5/1
  Delay5/1 -> Up Sample6/1, Delay6/1
  Delay6/1 -> Up Sample15/1
  X/1 -> Up Sample2/1, Delay/1

== system rate_change_filters_txrx_2ch/Tx Path/2-Ch Interp B/Sample RAMs/Delays ==
  X : Inport
  Delay{,1..6} (7 alike) : xbsIndex_r4/Delay  rst=off  infoeditControl=Selection of Reset will increase slice count due to use of real FFs and instead of SRLs  en=off  latency=1  dbl_ovrd=off  reg_retiming=off  block_type=delay
      settings: xl_area=[8 16 0 0 0 0 0]
  Up Sample{1..6,10,15} (8 alike) : xbsIndex_r4/Up Sample  sample_ratio=4  copy_samples=on  en=off  latency=0  dbl_ovrd=off  block_type=usamp
      settings: infoedit="Up samples input data.  Inserted values  can be zeros or copies of the most recent input sample.<P><P>Hardware notes: No hardware is needed if inserted values are copies of the input sample; otherwise, a mux and single bit flip-flop are used."  xl_area=[0 0 0 0 0 0 0]  block_version=10.1.3
  Out1 : Outport
  Out2 : Outport  Port=2
  Out3 : Outport  Port=3
  Out4 : Outport  Port=4
  Out5 : Outport  Port=5
  Out6 : Outport  Port=6
  Out7 : Outport  Port=7
  Out8 : Outport  Port=8
  wires:
  Up Sample15/1 -> Out8/1
  Up Sample6/1 -> Out7/1
  Up Sample5/1 -> Out6/1
  Up Sample4/1 -> Out5/1
  Up Sample3/1 -> Out4/1
  Up Sample10/1 -> Out3/1
  Up Sample1/1 -> Out2/1
  Up Sample2/1 -> Out1/1
  Delay/1 -> Up Sample1/1, Delay1/1
  Delay1/1 -> Up Sample10/1, Delay2/1
  Delay2/1 -> Up Sample3/1, Delay3/1
  Delay3/1 -> Up Sample4/1, Delay4/1
  Delay4/1 -> Up Sample5/1, Delay5/1
  Delay5/1 -> Up Sample6/1, Delay6/1
  Delay6/1 -> Up Sample15/1
  X/1 -> Up Sample2/1, Delay/1

== system rate_change_filters_txrx_2ch/Tx Path/2-Ch Interp B/Sample RAMs/Delays1 ==
  X : Inport
  Delay{,1..6} (7 alike) : xbsIndex_r4/Delay  rst=off  infoeditControl=Selection of Reset will increase slice count due to use of real FFs and instead of SRLs  en=off  latency=1  dbl_ovrd=off  reg_retiming=off  block_type=delay
      settings: xl_area=[8 16 0 0 0 0 0]
  Up Sample{1..6,10,15} (8 alike) : xbsIndex_r4/Up Sample  sample_ratio=4  copy_samples=on  en=off  latency=0  dbl_ovrd=off  block_type=usamp
      settings: infoedit="Up samples input data.  Inserted values  can be zeros or copies of the most recent input sample.<P><P>Hardware notes: No hardware is needed if inserted values are copies of the input sample; otherwise, a mux and single bit flip-flop are used."  xl_area=[0 0 0 0 0 0 0]  block_version=10.1.3
  Out1 : Outport
  Out2 : Outport  Port=2
  Out3 : Outport  Port=3
  Out4 : Outport  Port=4
  Out5 : Outport  Port=5
  Out6 : Outport  Port=6
  Out7 : Outport  Port=7
  Out8 : Outport  Port=8
  wires:
  X/1 -> Delay/1, Up Sample2/1
  Delay6/1 -> Up Sample15/1
  Delay5/1 -> Delay6/1, Up Sample6/1
  Delay4/1 -> Delay5/1, Up Sample5/1
  Delay3/1 -> Delay4/1, Up Sample4/1
  Delay2/1 -> Delay3/1, Up Sample3/1
  Delay1/1 -> Delay2/1, Up Sample10/1
  Delay/1 -> Delay1/1, Up Sample1/1
  Up Sample2/1 -> Out1/1
  Up Sample1/1 -> Out2/1
  Up Sample10/1 -> Out3/1
  Up Sample3/1 -> Out4/1
  Up Sample4/1 -> Out5/1
  Up Sample5/1 -> Out6/1
  Up Sample6/1 -> Out7/1
  Up Sample15/1 -> Out8/1

== system rate_change_filters_txrx_2ch/Rx Path/2-Ch Decimation A/Sample RAMs/MemoryA/TDD ==
  X : Inport
  TDD : xbsIndex_r4/Time Division Demultiplexer  frame_pattern=ones(1,4)  impl_style=Multiple Channel  vin=off  dbl_ovrd=off  explicit_period=off  period=1  block_type=tdd
      settings: infoedit=Samples presented at the input are selected and down-sampled according to the frame sampling pattern specified. The sampled input is presented either as a single or multiple channel at the output.  xl_area=[49 98 0 0 0 0 0]  block_version=9.1.01
  x[3] : Outport
  x[2] : Outport  Port=2
  x[1] : Outport  Port=3
  x[0] : Outport  Port=4
  wires:
  TDD/4 -> x[0]/1
  TDD/3 -> x[1]/1
  TDD/2 -> x[2]/1
  TDD/1 -> x[3]/1
  X/1 -> TDD/1

== system rate_change_filters_txrx_2ch/Rx Path/2-Ch Decimation A/Sample RAMs/MemoryB/TDD ==
  X : Inport
  TDD : xbsIndex_r4/Time Division Demultiplexer  frame_pattern=ones(1,4)  impl_style=Multiple Channel  vin=off  dbl_ovrd=off  explicit_period=off  period=1  block_type=tdd
      settings: infoedit=Samples presented at the input are selected and down-sampled according to the frame sampling pattern specified. The sampled input is presented either as a single or multiple channel at the output.  xl_area=[49 98 0 0 0 0 0]  block_version=9.1.01
  x[3] : Outport
  x[2] : Outport  Port=2
  x[1] : Outport  Port=3
  x[0] : Outport  Port=4
  wires:
  X/1 -> TDD/1
  TDD/1 -> x[3]/1
  TDD/2 -> x[2]/1
  TDD/3 -> x[1]/1
  TDD/4 -> x[0]/1

== system rate_change_filters_txrx_2ch/Rx Path/2-Ch Decimation B/Sample RAMs/MemoryA/TDD ==
  X : Inport
  TDD : xbsIndex_r4/Time Division Demultiplexer  frame_pattern=ones(1,4)  impl_style=Multiple Channel  vin=off  dbl_ovrd=off  explicit_period=off  period=1  block_type=tdd
      settings: infoedit=Samples presented at the input are selected and down-sampled according to the frame sampling pattern specified. The sampled input is presented either as a single or multiple channel at the output.  xl_area=[49 98 0 0 0 0 0]  block_version=9.1.01
  x[3] : Outport
  x[2] : Outport  Port=2
  x[1] : Outport  Port=3
  x[0] : Outport  Port=4
  wires:
  X/1 -> TDD/1
  TDD/1 -> x[3]/1
  TDD/2 -> x[2]/1
  TDD/3 -> x[1]/1
  TDD/4 -> x[0]/1

== system rate_change_filters_txrx_2ch/Rx Path/2-Ch Decimation B/Sample RAMs/MemoryB/TDD ==
  X : Inport
  TDD : xbsIndex_r4/Time Division Demultiplexer  frame_pattern=ones(1,4)  impl_style=Multiple Channel  vin=off  dbl_ovrd=off  explicit_period=off  period=1  block_type=tdd
      settings: infoedit=Samples presented at the input are selected and down-sampled according to the frame sampling pattern specified. The sampled input is presented either as a single or multiple channel at the output.  xl_area=[49 98 0 0 0 0 0]  block_version=9.1.01
  x[3] : Outport
  x[2] : Outport  Port=2
  x[1] : Outport  Port=3
  x[0] : Outport  Port=4
  wires:
  TDD/4 -> x[0]/1
  TDD/3 -> x[1]/1
  TDD/2 -> x[2]/1
  TDD/1 -> x[3]/1
  X/1 -> TDD/1
